simulink model "Exercise_29"  (R2023a)
settings: Solver=VariableStepAuto  StartTime=0.0  StopTime=10.0  RelTol=1e-3
settings Model: Creator=Admin  LastModifiedBy=Admin

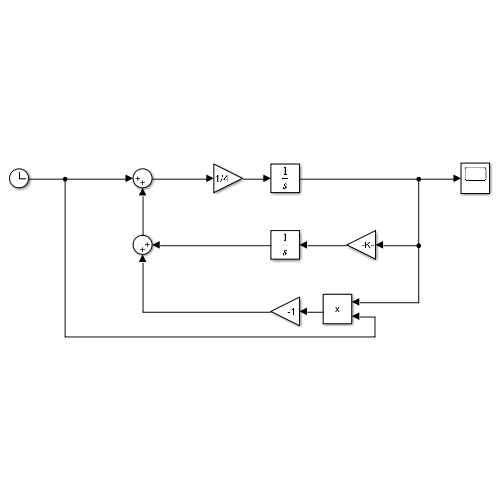
[thumbnail: Simulink's stored preview of the top-level diagram]
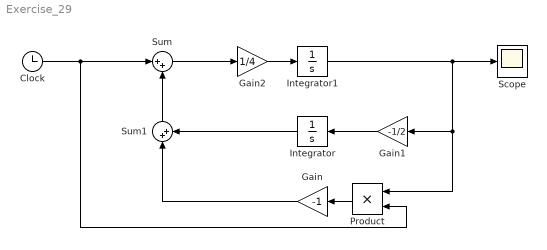
== system Exercise_29 ==
  Clock : Clock
  Gain : Gain  Gain=-1
  Gain1 : Gain  Gain=-1/2
  Gain2 : Gain  Gain=1/4
  Integrator : Integrator
  Integrator1 : Integrator
  Product : Product
  Scope : Scope
  Sum : Sum  Inputs=|++
  Sum1 : Sum  Inputs=|++
  wires:
  Clock/1 -> Product/2, Sum/1
  Gain1/1 -> Integrator/1
  Gain2/1 -> Integrator1/1
  Sum/1 -> Gain2/1
  Integrator/1 -> Sum1/2
  Product/1 -> Gain/1
  Gain/1 -> Sum1/1
  Sum1/1 -> Sum/2
  Integrator1/1 -> Product/1, Gain1/1, Scope/1
